simulink model "dc_motor"  (R2021a)
settings: Solver=FixedStepAuto  StartTime=0.0  StopTime=100.0  FixedStep=0.001  RelTol=1e-3
values from neighbouring files (symbols this model uses):
  dm = 0.1    [Params.m]
  J = 0.005332    [Params.m]
  Kd = 0.4    [Params.m]
  Ki = 0    [Params.m]
  Km = 10    [Params.m]
  Kp = 60    [Params.m]
  sat = inf    [Params.m]
undefined symbols (not defined in the file or in its folder): DiscIntNeverNeededParam
libraries: simulink x3
settings Model: Creator=antoninoparisi  LastModifiedBy=antoninoparisi
settings SolverCC: AlgebraicLoopSolver=TrustRegion
settings DebuggingCC: SFMachineParentedDataDiag=warning

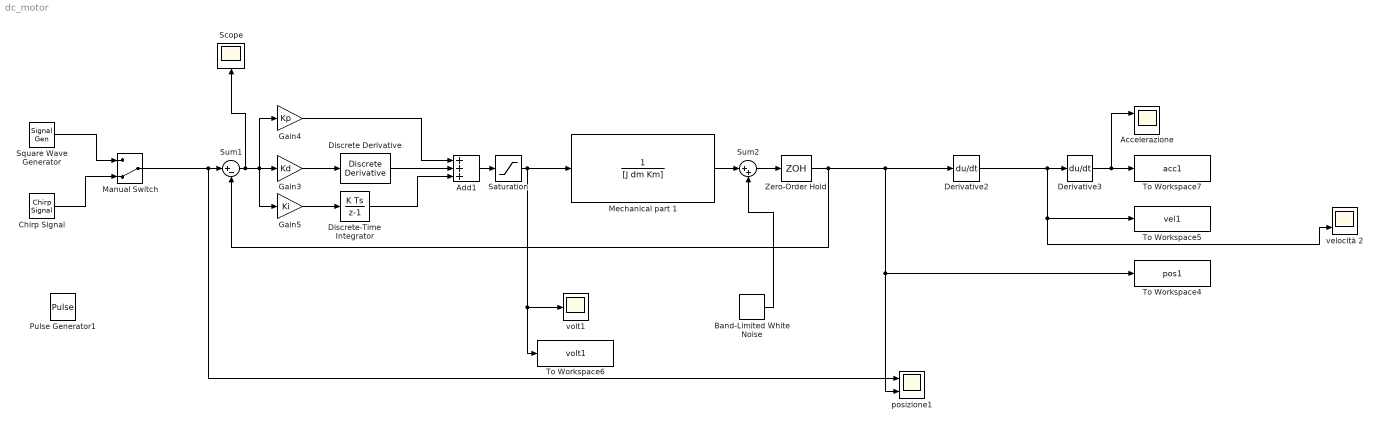
== system dc_motor ==
  "Accelerazione " : Scope  NumInputPorts=2
  Add1 : Sum  Inputs=+++
  Band-Limited White Noise : simulink/Sources/Band-Limited White Noise  Cov=[0.000000005]  Ts=0.001  seed=[23341]
  Chirp Signal : simulink/Sources/Chirp Signal  f1=0.1  T=100  f2=10
  Derivative2 : Derivative
  Derivative3 : Derivative
  Discrete Derivative : simulink/Discrete/Discrete Derivative  gainval=1.0  ICPrevScaledInput=0.0  OutMin=[]  OutMax=[]  OutDataType=fixdt(1, 16)  OutScaling=2^-10  DoSatur=off
  Discrete-Time Integrator : DiscreteIntegrator  SampleTime=-1  ICPrevOutput=DiscIntNeverNeededParam  ICPrevScaledInput=DiscIntNeverNeededParam
  Gain3 : Gain  Gain=Kd
  Gain4 : Gain  Gain=Kp
  Gain5 : Gain  Gain=Ki
  Manual Switch : ManualSwitch  CurrentSetting=0
  Mechanical part 1 : TransferFcn  Denominator=[J dm Km]
  Pulse Generator1 : DiscretePulseGenerator  PulseType=Time based  Period=10  PulseWidth=5
  Saturation : Saturate  UpperLimit=sat  LowerLimit=-sat
  Scope : Scope
  Square Wave Generator : SignalGenerator  WaveForm=square  Amplitude=0.3  Units=rad/sec
  Sum1 : Sum  Inputs=|+-
  Sum2 : Sum  Inputs=|++
  To Workspace4 : ToWorkspace  VariableName=pos1  SaveFormat=Timeseries  SampleTime=-1
  To Workspace5 : ToWorkspace  VariableName=vel1  SaveFormat=Timeseries  SampleTime=-1
  To Workspace6 : ToWorkspace  VariableName=volt1  SaveFormat=Timeseries  SampleTime=-1
  To Workspace7 : ToWorkspace  VariableName=acc1  SaveFormat=Timeseries  SampleTime=-1
  Zero-Order Hold : ZeroOrderHold  SampleTime=-1
  posizione1 : Scope  NumInputPorts=2
  velocità 2 : Scope  NumInputPorts=2
  volt1 : Scope
  wires:
  Gain5/1 -> Discrete-Time Integrator/1
  Gain4/1 -> Add1/1
  Discrete-Time Integrator/1 -> Add1/3
  Sum1/1 -> Scope/1, Gain5/1, Gain4/1, Gain3/1
  Zero-Order Hold/1 -> Sum1/2, posizione1/2, To Workspace4/1, Derivative2/1
  Discrete Derivative/1 -> Add1/2
  Gain3/1 -> Discrete Derivative/1
  Add1/1 -> Saturation/1
  Saturation/1 -> Mechanical part 1/1, To Workspace6/1, volt1/1
  Square Wave Generator/1 -> Manual Switch/1
  Chirp Signal/1 -> Manual Switch/2
  Mechanical part 1/1 -> Sum2/1
  Sum2/1 -> Zero-Order Hold/1
  Manual Switch/1 -> posizione1/1, Sum1/1
  Derivative2/1 -> Derivative3/1, velocità 2/2, To Workspace5/1
  Derivative3/1 -> "Accelerazione "/1, To Workspace7/1
  Band-Limited White Noise/1 -> Sum2/2
